simulink model "filter_demo"  (Simulink 7.1)
settings: Solver=ode45  StartTime=0.0  StopTime=10.0  RelTol=1e-3
libraries: simulink x1
settings Model: Creator=minakata  LastModifiedBy=minakata

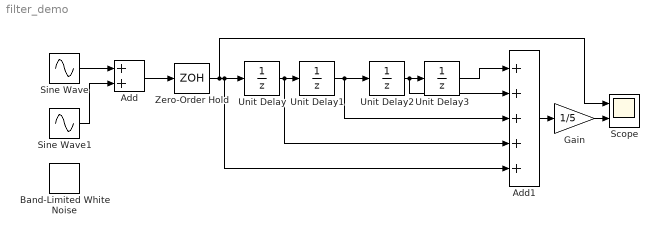
== system filter_demo ==
  Add : Sum  OutDataType=sfix(16)  OutScaling=2^-10
  Add1 : Sum  Inputs=+++++  OutDataType=sfix(16)  OutScaling=2^-10
  Band-Limited White Noise : simulink/Sources/Band-Limited White Noise  SystemSampleTime=-1  Cov=[0.1]  Ts=0.01  seed=[23341]
  Gain : Gain  Gain=1/5  ParameterDataType=sfix(16)  ParameterScaling=2^0  OutDataType=sfix(16)  OutScaling=2^0
  Scope : Scope  NumInputPorts=2
      settings: YMin=-5~-5  YMax=5~5
  Sine Wave : Sin  Amplitude=10  Frequency=0.25*2*pi  SampleTime=0
  Sine Wave1 : Sin  Frequency=30*2*pi  SampleTime=0
  Unit Delay{,1..3} (4 alike) : UnitDelay  SampleTime=-1
  Zero-Order Hold : ZeroOrderHold  SampleTime=0.01
  wires:
  Sine Wave/1 -> Add/1
  Add/1 -> Zero-Order Hold/1
  Add1/1 -> Gain/1
  Zero-Order Hold/1 -> Unit Delay/1, Add1/5, Scope/1
  Gain/1 -> Scope/2
  Unit Delay3/1 -> Add1/1
  Unit Delay2/1 -> Unit Delay3/1, Add1/2
  Unit Delay1/1 -> Unit Delay2/1, Add1/3
  Unit Delay/1 -> Unit Delay1/1, Add1/4
  Sine Wave1/1 -> Add/2
